simulink model "ES259A_BattVltgCorrln"  (R2013b)
settings: Solver=FixedStepDiscrete  SolverMode=SingleTasking  StartTime=0.0  StopTime=Inf  FixedStep=0.002  RelTol=1e-3
values from neighbouring files (symbols this model uses):
  BattVltgCorrlnAllwdVltgDif = DataDict.Calibration    [ES259A_BattVltgCorrln_DataDict.m]
  BattVltgCorrlnBattLoVltg = DataDict.Calibration    [ES259A_BattVltgCorrln_DataDict.m]
  BattVltgCorrlnBattOverVltg = DataDict.Calibration    [ES259A_BattVltgCorrln_DataDict.m]
  BattVltgCorrlnBattUnderVltg = DataDict.Calibration    [ES259A_BattVltgCorrln_DataDict.m]
  BattVltgCorrlnNtc0x03C0x0440x04CFailStep = DataDict.Calibration    [ES259A_BattVltgCorrln_DataDict.m]
  BattVltgCorrlnNtc0x03C0x0440x04CPassStep = DataDict.Calibration    [ES259A_BattVltgCorrln_DataDict.m]
  BattVltgCorrlnNtc0x03DFailStep = DataDict.Calibration    [ES259A_BattVltgCorrln_DataDict.m]
  BattVltgCorrlnNtc0x03DPassStep = DataDict.Calibration    [ES259A_BattVltgCorrln_DataDict.m]
  BattVltgCorrlnNtc0x0B0FailStep = DataDict.Calibration    [ES259A_BattVltgCorrln_DataDict.m]
  BattVltgCorrlnNtc0x0B0PassStep = DataDict.Calibration    [ES259A_BattVltgCorrln_DataDict.m]
  BattVltgCorrlnNtc0x0B1FailStep = DataDict.Calibration    [ES259A_BattVltgCorrln_DataDict.m]
  BattVltgCorrlnNtc0x0B1PassStep = DataDict.Calibration    [ES259A_BattVltgCorrln_DataDict.m]
  BattVltgCorrlnNtc0x0B5FailStep = DataDict.Calibration    [ES259A_BattVltgCorrln_DataDict.m]
  BattVltgCorrlnNtc0x0B5PassStep = DataDict.Calibration    [ES259A_BattVltgCorrln_DataDict.m]
  BattVltgCorrlnRcvrlBattLoVltg = DataDict.Calibration    [ES259A_BattVltgCorrln_DataDict.m]
  BattVltgCorrlnRcvrlBattOverVltg = DataDict.Calibration    [ES259A_BattVltgCorrln_DataDict.m]
  BattVltgCorrlnRcvrlBattUnderVltg = DataDict.Calibration    [ES259A_BattVltgCorrln_DataDict.m]
  BattVltgCorrlnSysMinVltg = DataDict.ImprtdCal    [ES250A_BattVltg_DataDict.m]    (also in ES259A_BattVltgCorrln_DataDict.m = DataDict.Calibration)
  BattVltgSwdMax = DataDict.Calibration    [ES250A_BattVltg_DataDict.m]
  ELECGLBPRM_STRTUPSTPWRDISCNCTBTESTCMPL_CNT_U08 = DataDict.Constant    [ES999A_ElecGlbPrm_DataDict.m]
  SYSVLTGFLTDUALIVTR_CNT_U08 = DataDict.Constant    [ES259A_BattVltgCorrln_DataDict.m]
undefined symbols (not defined in the file or in its folder): NtcNr1, NtcSts1, SigQlfr1
libraries: simulink x14
(part 6 of 7)

== system ES259A_BattVltgCorrln/BattVltgCorrln/BattVltgCorrlnPer1/WarmInit or Enable/Determine Independent Signals/Diagnose Inputs/NTC 3D/Pass NTC 3D/Copyright1 ==

== system ES259A_BattVltgCorrln/BattVltgCorrln/BattVltgCorrlnPer1/WarmInit or Enable/Determine Independent Signals/Diagnose Inputs/NTC 3D/Pass NTC 3D/SetNtcSts ==
  note: Only pass values 2 or 3 as input to NtcSts.
      | 2: PrePassd
      | 3: PreFaild
  NtcNr : Inport
  NtcStInfo : Inport  Port=2
  NtcSts : Inport  Port=3
  DebStep : Inport  Port=4
  Copyright1 : Subsystem  Description=|  mask(Copyright Information){none=on}
      | Copyright info block.                                               
      |                                                                     
      | Place copyright information at the top of every subsystem in design.
      mask prompts: none "No parameters"
      mask help: Place copyright information at the top of every subsystem in design.
      mask Display:
      | NxtrConf = 'Nexteer Confidential';
      | 
      | sys = bdroot; %handle for the current model ("system")
      | first = get_param(sys,'Created');
      | if(isempty(first))
      |     first = datestr(now,'yyyy');
      | else
      |     first = first(end-3:end);  %year is last four digits
      | end
      | 
      | last = get_param(sys,'LastModifiedDate');
      | if isempty(last)
      |     last = datestr(now,'yyyy');
      | else
      |     last = last(end-3:end);
      | end
      | 
      | if strcmp(first,last)
      |     fprintf('%s\nCopyright  %s Nexteer',NxtrConf,first);
      | else
      |     fprintf('%s\n%s%s-%s Nexteer',NxtrConf,char(169),first,last);
      | end
  Data Store Write1 : DataStoreWrite  RequirementInfo={} %GIDa_6d6848f0_15f2_42f8_b891_1052be6b64a1  DataStoreName=NtcQlfr3D
  ISO Fault Debounce Design NOT TO BE IMPLEMENTED IN THIS FDD USED ONLY FOR SIMULATION PURPOSES : Stateflow chart  TreatAsAtomicUnit=on
  Only here because I could not get model to run with enumerations in the stateflow diagram : DataTypeConversion  OutDataTypeStr=uint8
  Terminator : Terminator
  Terminator1 : Terminator
  wires:
  NtcStInfo/1 -> Terminator1/1
  NtcNr/1 -> Terminator/1
  NtcSts/1 -> Only here because I could not get model to run with enumerations in the stateflow diagram/1
  DebStep/1 -> ISO Fault Debounce Design NOT TO BE IMPLEMENTED IN THIS FDD USED ONLY FOR SIMULATION PURPOSES/2(DebStep)
  ISO Fault Debounce Design NOT TO BE IMPLEMENTED IN THIS FDD USED ONLY FOR SIMULATION PURPOSES/1(Qualifier) -> Data Store Write1/1
  Only here because I could not get model to run with enumerations in the stateflow diagram/1 -> ISO Fault Debounce Design NOT TO BE IMPLEMENTED IN THIS FDD USED ONLY FOR SIMULATION PURPOSES/1(NtcSts)

== system ES259A_BattVltgCorrln/BattVltgCorrln/BattVltgCorrlnPer1/WarmInit or Enable/Determine Independent Signals/Diagnose Inputs/NTC 44/GetNtcQlfrSts 0x044/Copyright1 ==

== system ES259A_BattVltgCorrln/BattVltgCorrln/BattVltgCorrlnPer1/WarmInit or Enable/Determine Independent Signals/Diagnose Inputs/NTC 44/GetNtcQlfrSts 0x044/GetNtcQlfrSts ==
  note: Enumeration of SigQlfr1
      |         SIGQLFR_NORES   (0)
      |         SIGQLFR_PASSD    (1)
      |         SIGQLFR_FAILD      (2)
  NtcNr : Inport
  CopyRight2 : Subsystem  Description=|  mask(Copyright Information){none=on}
      | Copyright info block.                                               
      |                                                                     
      | Place copyright information at the top of every subsystem in design.
      mask prompts: none "No parameters"
      mask help: Place copyright information at the top of every subsystem in design.
      mask Display:
      | NxtrConf = 'Nexteer Confidential';
      | 
      | sys = bdroot; %handle for the current model ("system")
      | first = get_param(sys,'Created');
      | first = first(end-3:end);  %year is last four digits
      | 
      | last = get_param(sys,'LastModifiedDate');
      | if isempty(last)
      |     last = datestr(now,'yyyy');
      | else
      |     last = last(end-3:end);
      | end
      | 
      | if strcmp(first,last)
      |     fprintf('%s -- Copyright %s Nexteer',NxtrConf,first)
      | else
      |     fprintf('%s -- %s%s- %s Nexteer',NxtrConf,char(169),first,last)
      | end
  Data Store Read5 : DataStoreRead  DataStoreName=NtcQlfr44
  Data Type Conversion : DataTypeConversion  OutDataTypeStr=uint8
  EOK : Constant  OutDataTypeStr=uint8
  Terminator : Terminator
  Return : Outport  InitialOutput=1
  Ntc0x044QlfrSts : Outport  Port=2
  wires:
  Data Store Read5/1 -> Data Type Conversion/1
  EOK/1 -> Return/1
  NtcNr/1 -> Terminator/1
  Data Type Conversion/1 -> Ntc0x044QlfrSts/1

== system ES259A_BattVltgCorrln/BattVltgCorrln/BattVltgCorrlnPer1/WarmInit or Enable/Determine Independent Signals/Diagnose Inputs/NTC 44/SetNtcSts 0x044/Copyright1 ==

== system ES259A_BattVltgCorrln/BattVltgCorrln/BattVltgCorrlnPer1/WarmInit or Enable/Determine Independent Signals/Diagnose Inputs/NTC 44/SetNtcSts 0x044/Do Nothing ==
  Action Port : ActionPort  ActionType=then
  Copyright1 : Subsystem  Description=|  mask(Copyright Information){none=on}
      | Copyright info block.                                               
      |                                                                     
      | Place copyright information at the top of every subsystem in design.
      mask prompts: none "No parameters"
      mask help: Place copyright information at the top of every subsystem in design.
      mask Display:
      | NxtrConf = 'Nexteer Confidential';
      | 
      | sys = bdroot; %handle for the current model ("system")
      | first = get_param(sys,'Created');
      | if(isempty(first))
      |     first = datestr(now,'yyyy');
      | else
      |     first = first(end-3:end);  %year is last four digits
      | end
      | 
      | last = get_param(sys,'LastModifiedDate');
      | if isempty(last)
      |     last = datestr(now,'yyyy');
      | else
      |     last = last(end-3:end);
      | end
      | 
      | if strcmp(first,last)
      |     fprintf('%s\nCopyright  %s Nexteer',NxtrConf,first);
      | else
      |     fprintf('%s\n%s%s-%s Nexteer',NxtrConf,char(169),first,last);
      | end

== system ES259A_BattVltgCorrln/BattVltgCorrln/BattVltgCorrlnPer1/WarmInit or Enable/Determine Independent Signals/Diagnose Inputs/NTC 44/SetNtcSts 0x044/Fails the test ==
  Action Port : ActionPort  ActionType=else
  BattVltgCorrlnNtc0x044FailStep : Constant  Value=BattVltgCorrlnNtc0x03C0x0440x04CFailStep
  Copyright1 : Subsystem  Description=|  mask(Copyright Information){none=on}
      | Copyright info block.                                               
      |                                                                     
      | Place copyright information at the top of every subsystem in design.
      mask prompts: none "No parameters"
      mask help: Place copyright information at the top of every subsystem in design.
      mask Display:
      | NxtrConf = 'Nexteer Confidential';
      | 
      | sys = bdroot; %handle for the current model ("system")
      | first = get_param(sys,'Created');
      | if(isempty(first))
      |     first = datestr(now,'yyyy');
      | else
      |     first = first(end-3:end);  %year is last four digits
      | end
      | 
      | last = get_param(sys,'LastModifiedDate');
      | if isempty(last)
      |     last = datestr(now,'yyyy');
      | else
      |     last = last(end-3:end);
      | end
      | 
      | if strcmp(first,last)
      |     fprintf('%s\nCopyright  %s Nexteer',NxtrConf,first);
      | else
      |     fprintf('%s\n%s%s-%s Nexteer',NxtrConf,char(169),first,last);
      | end
  Parameter Byte : Constant  OutDataTypeStr=uint8
  Status Type : Constant  Value=NtcSts1.NTCSTS_PREFAILD
  Ntc0x044 NtcStInfo : Outport
  Ntc0x044 NtcSts : Outport  Port=2
  Ntc0x044 FailStep : Outport  Port=3
  wires:
  Status Type/1 -> Ntc0x044 NtcSts/1
  BattVltgCorrlnNtc0x044FailStep/1 -> Ntc0x044 FailStep/1
  Parameter Byte/1 -> Ntc0x044 NtcStInfo/1

== system ES259A_BattVltgCorrln/BattVltgCorrln/BattVltgCorrlnPer1/WarmInit or Enable/Determine Independent Signals/Diagnose Inputs/NTC 44/SetNtcSts 0x044/Passes the test ==
  Action Port : ActionPort  ActionType=elseif
  BattVltgCorrlnNtc0x044PassStep : Constant  Value=BattVltgCorrlnNtc0x03C0x0440x04CPassStep
  Copyright1 : Subsystem  Description=|  mask(Copyright Information){none=on}
      | Copyright info block.                                               
      |                                                                     
      | Place copyright information at the top of every subsystem in design.
      mask prompts: none "No parameters"
      mask help: Place copyright information at the top of every subsystem in design.
      mask Display:
      | NxtrConf = 'Nexteer Confidential';
      | 
      | sys = bdroot; %handle for the current model ("system")
      | first = get_param(sys,'Created');
      | if(isempty(first))
      |     first = datestr(now,'yyyy');
      | else
      |     first = first(end-3:end);  %year is last four digits
      | end
      | 
      | last = get_param(sys,'LastModifiedDate');
      | if isempty(last)
      |     last = datestr(now,'yyyy');
      | else
      |     last = last(end-3:end);
      | end
      | 
      | if strcmp(first,last)
      |     fprintf('%s\nCopyright  %s Nexteer',NxtrConf,first);
      | else
      |     fprintf('%s\n%s%s-%s Nexteer',NxtrConf,char(169),first,last);
      | end
  Parameter Byte Data1 : Constant  Value=0  OutDataTypeStr=uint8
  Status Type : Constant  Value=NtcSts1.NTCSTS_PREPASSD
  Ntc0x044 NtcStInfo : Outport
  Ntc0x044 NtcSts : Outport  Port=2
  Ntc0x044 PassStep : Outport  Port=3
  wires:
  Status Type/1 -> Ntc0x044 NtcSts/1
  BattVltgCorrlnNtc0x044PassStep/1 -> Ntc0x044 PassStep/1
  Parameter Byte Data1/1 -> Ntc0x044 NtcStInfo/1

== system ES259A_BattVltgCorrln/BattVltgCorrln/BattVltgCorrlnPer1/WarmInit or Enable/Determine Independent Signals/Diagnose Inputs/NTC 44/SetNtcSts 0x044/SetNtcSts ==
  note: Only pass values 2 or 3 as input to NtcSts.
      | 2: PrePassd
      | 3: PreFaild
  NtcNr : Inport
  NtcStInfo : Inport  Port=2
  NtcSts : Inport  Port=3
  DebStep : Inport  Port=4
  Copyright1 : Subsystem  Description=|  mask(Copyright Information){none=on}
      | Copyright info block.                                               
      |                                                                     
      | Place copyright information at the top of every subsystem in design.
      mask prompts: none "No parameters"
      mask help: Place copyright information at the top of every subsystem in design.
      mask Display:
      | NxtrConf = 'Nexteer Confidential';
      | 
      | sys = bdroot; %handle for the current model ("system")
      | first = get_param(sys,'Created');
      | if(isempty(first))
      |     first = datestr(now,'yyyy');
      | else
      |     first = first(end-3:end);  %year is last four digits
      | end
      | 
      | last = get_param(sys,'LastModifiedDate');
      | if isempty(last)
      |     last = datestr(now,'yyyy');
      | else
      |     last = last(end-3:end);
      | end
      | 
      | if strcmp(first,last)
      |     fprintf('%s\nCopyright  %s Nexteer',NxtrConf,first);
      | else
      |     fprintf('%s\n%s%s-%s Nexteer',NxtrConf,char(169),first,last);
      | end
  Data Store Write1 : DataStoreWrite  RequirementInfo={} %GIDa_89fda807_da4f_4ef8_9f7d_e78b25b40171  DataStoreName=NtcQlfr44
  ISO Fault Debounce Design NOT TO BE IMPLEMENTED IN THIS FDD USED ONLY FOR SIMULATION PURPOSES : Stateflow chart  TreatAsAtomicUnit=on
  Only here because I could not get model to run with enumerations in the stateflow diagram : DataTypeConversion  OutDataTypeStr=uint8
  Terminator : Terminator
  Terminator1 : Terminator
  wires:
  NtcStInfo/1 -> Terminator1/1
  NtcNr/1 -> Terminator/1
  NtcSts/1 -> Only here because I could not get model to run with enumerations in the stateflow diagram/1
  DebStep/1 -> ISO Fault Debounce Design NOT TO BE IMPLEMENTED IN THIS FDD USED ONLY FOR SIMULATION PURPOSES/2(DebStep)
  Only here because I could not get model to run with enumerations in the stateflow diagram/1 -> ISO Fault Debounce Design NOT TO BE IMPLEMENTED IN THIS FDD USED ONLY FOR SIMULATION PURPOSES/1(NtcSts)
  ISO Fault Debounce Design NOT TO BE IMPLEMENTED IN THIS FDD USED ONLY FOR SIMULATION PURPOSES/1(Qualifier) -> Data Store Write1/1

== system ES259A_BattVltgCorrln/BattVltgCorrln/BattVltgCorrlnPer1/WarmInit or Enable/Determine Independent Signals/Diagnose Inputs/NTC 4C/GetNtcQlfrSts 0x04C/Copyright1 ==

== system ES259A_BattVltgCorrln/BattVltgCorrln/BattVltgCorrlnPer1/WarmInit or Enable/Determine Independent Signals/Diagnose Inputs/NTC 4C/GetNtcQlfrSts 0x04C/GetNtcQlfrSts ==
  note: Enumeration of SigQlfr1
      |         SIGQLFR_NORES   (0)
      |         SIGQLFR_PASSD    (1)
      |         SIGQLFR_FAILD      (2)
  NtcNr : Inport
  CopyRight2 : Subsystem  Description=|  mask(Copyright Information){none=on}
      | Copyright info block.                                               
      |                                                                     
      | Place copyright information at the top of every subsystem in design.
      mask prompts: none "No parameters"
      mask help: Place copyright information at the top of every subsystem in design.
      mask Display:
      | NxtrConf = 'Nexteer Confidential';
      | 
      | sys = bdroot; %handle for the current model ("system")
      | first = get_param(sys,'Created');
      | first = first(end-3:end);  %year is last four digits
      | 
      | last = get_param(sys,'LastModifiedDate');
      | if isempty(last)
      |     last = datestr(now,'yyyy');
      | else
      |     last = last(end-3:end);
      | end
      | 
      | if strcmp(first,last)
      |     fprintf('%s -- Copyright %s Nexteer',NxtrConf,first)
      | else
      |     fprintf('%s -- %s%s- %s Nexteer',NxtrConf,char(169),first,last)
      | end
  Data Store Read5 : DataStoreRead  DataStoreName=NtcQlfr4C
  Data Type Conversion : DataTypeConversion  OutDataTypeStr=uint8
  EOK : Constant  OutDataTypeStr=uint8
  Terminator : Terminator
  Return : Outport  InitialOutput=1
  Ntc0x04CQlfrSts : Outport  Port=2
  wires:
  Data Store Read5/1 -> Data Type Conversion/1
  EOK/1 -> Return/1
  NtcNr/1 -> Terminator/1
  Data Type Conversion/1 -> Ntc0x04CQlfrSts/1

== system ES259A_BattVltgCorrln/BattVltgCorrln/BattVltgCorrlnPer1/WarmInit or Enable/Determine Independent Signals/Diagnose Inputs/NTC 4C/SetNtcSts 0x04C/Copyright1 ==

== system ES259A_BattVltgCorrln/BattVltgCorrln/BattVltgCorrlnPer1/WarmInit or Enable/Determine Independent Signals/Diagnose Inputs/NTC 4C/SetNtcSts 0x04C/Do Nothing ==
  Action Port : ActionPort  ActionType=then
  Copyright1 : Subsystem  Description=|  mask(Copyright Information){none=on}
      | Copyright info block.                                               
      |                                                                     
      | Place copyright information at the top of every subsystem in design.
      mask prompts: none "No parameters"
      mask help: Place copyright information at the top of every subsystem in design.
      mask Display:
      | NxtrConf = 'Nexteer Confidential';
      | 
      | sys = bdroot; %handle for the current model ("system")
      | first = get_param(sys,'Created');
      | if(isempty(first))
      |     first = datestr(now,'yyyy');
      | else
      |     first = first(end-3:end);  %year is last four digits
      | end
      | 
      | last = get_param(sys,'LastModifiedDate');
      | if isempty(last)
      |     last = datestr(now,'yyyy');
      | else
      |     last = last(end-3:end);
      | end
      | 
      | if strcmp(first,last)
      |     fprintf('%s\nCopyright  %s Nexteer',NxtrConf,first);
      | else
      |     fprintf('%s\n%s%s-%s Nexteer',NxtrConf,char(169),first,last);
      | end

== system ES259A_BattVltgCorrln/BattVltgCorrln/BattVltgCorrlnPer1/WarmInit or Enable/Determine Independent Signals/Diagnose Inputs/NTC 4C/SetNtcSts 0x04C/Fails the test ==
  Action Port : ActionPort  ActionType=else
  BattVltgCorrlnNtc0x04CFailStep : Constant  Value=BattVltgCorrlnNtc0x03C0x0440x04CFailStep
  Copyright1 : Subsystem  Description=|  mask(Copyright Information){none=on}
      | Copyright info block.                                               
      |                                                                     
      | Place copyright information at the top of every subsystem in design.
      mask prompts: none "No parameters"
      mask help: Place copyright information at the top of every subsystem in design.
      mask Display:
      | NxtrConf = 'Nexteer Confidential';
      | 
      | sys = bdroot; %handle for the current model ("system")
      | first = get_param(sys,'Created');
      | if(isempty(first))
      |     first = datestr(now,'yyyy');
      | else
      |     first = first(end-3:end);  %year is last four digits
      | end
      | 
      | last = get_param(sys,'LastModifiedDate');
      | if isempty(last)
      |     last = datestr(now,'yyyy');
      | else
      |     last = last(end-3:end);
      | end
      | 
      | if strcmp(first,last)
      |     fprintf('%s\nCopyright  %s Nexteer',NxtrConf,first);
      | else
      |     fprintf('%s\n%s%s-%s Nexteer',NxtrConf,char(169),first,last);
      | end
  Parameter Byte : Constant  OutDataTypeStr=uint8
  Status Type : Constant  Value=NtcSts1.NTCSTS_PREFAILD
  Ntc0x04C NtcStInfo : Outport
  Ntc0x04C NtcSts : Outport  Port=2
  Ntc0x04C PassStep : Outport  Port=3
  wires:
  Status Type/1 -> Ntc0x04C NtcSts/1
  Parameter Byte/1 -> Ntc0x04C NtcStInfo/1
  BattVltgCorrlnNtc0x04CFailStep/1 -> Ntc0x04C PassStep/1

== system ES259A_BattVltgCorrln/BattVltgCorrln/BattVltgCorrlnPer1/WarmInit or Enable/Determine Independent Signals/Diagnose Inputs/NTC 4C/SetNtcSts 0x04C/Passes the test ==
  Action Port : ActionPort  ActionType=elseif
  BattVltgCorrlnNtc0x04CPassStep : Constant  Value=BattVltgCorrlnNtc0x03C0x0440x04CPassStep
  Copyright1 : Subsystem  Description=|  mask(Copyright Information){none=on}
      | Copyright info block.                                               
      |                                                                     
      | Place copyright information at the top of every subsystem in design.
      mask prompts: none "No parameters"
      mask help: Place copyright information at the top of every subsystem in design.
      mask Display:
      | NxtrConf = 'Nexteer Confidential';
      | 
      | sys = bdroot; %handle for the current model ("system")
      | first = get_param(sys,'Created');
      | if(isempty(first))
      |     first = datestr(now,'yyyy');
      | else
      |     first = first(end-3:end);  %year is last four digits
      | end
      | 
      | last = get_param(sys,'LastModifiedDate');
      | if isempty(last)
      |     last = datestr(now,'yyyy');
      | else
      |     last = last(end-3:end);
      | end
      | 
      | if strcmp(first,last)
      |     fprintf('%s\nCopyright  %s Nexteer',NxtrConf,first);
      | else
      |     fprintf('%s\n%s%s-%s Nexteer',NxtrConf,char(169),first,last);
      | end
  Parameter Byte Data1 : Constant  Value=0  OutDataTypeStr=uint8
  Status Type : Constant  Value=NtcSts1.NTCSTS_PREPASSD
  Ntc0x04C NtcStInfo : Outport
  Ntc0x04C NtcSts : Outport  Port=2
  Ntc0x04C PassStep : Outport  Port=3
  wires:
  Status Type/1 -> Ntc0x04C NtcSts/1
  Parameter Byte Data1/1 -> Ntc0x04C NtcStInfo/1
  BattVltgCorrlnNtc0x04CPassStep/1 -> Ntc0x04C PassStep/1

== system ES259A_BattVltgCorrln/BattVltgCorrln/BattVltgCorrlnPer1/WarmInit or Enable/Determine Independent Signals/Diagnose Inputs/NTC 4C/SetNtcSts 0x04C/SetNtcSts ==
  note: Only pass values 2 or 3 as input to NtcSts.
      | 2: PrePassd
      | 3: PreFaild
  NtcNr : Inport
  NtcStInfo : Inport  Port=2
  NtcSts : Inport  Port=3
  DebStep : Inport  Port=4
  Copyright1 : Subsystem  Description=|  mask(Copyright Information){none=on}
      | Copyright info block.                                               
      |                                                                     
      | Place copyright information at the top of every subsystem in design.
      mask prompts: none "No parameters"
      mask help: Place copyright information at the top of every subsystem in design.
      mask Display:
      | NxtrConf = 'Nexteer Confidential';
      | 
      | sys = bdroot; %handle for the current model ("system")
      | first = get_param(sys,'Created');
      | if(isempty(first))
      |     first = datestr(now,'yyyy');
      | else
      |     first = first(end-3:end);  %year is last four digits
      | end
      | 
      | last = get_param(sys,'LastModifiedDate');
      | if isempty(last)
      |     last = datestr(now,'yyyy');
      | else
      |     last = last(end-3:end);
      | end
      | 
      | if strcmp(first,last)
      |     fprintf('%s\nCopyright  %s Nexteer',NxtrConf,first);
      | else
      |     fprintf('%s\n%s%s-%s Nexteer',NxtrConf,char(169),first,last);
      | end
  Data Store Write1 : DataStoreWrite  RequirementInfo={} %GIDa_0b6832db_b5ce_44a6_8c80_102ac06d195d  DataStoreName=NtcQlfr4C
  ISO Fault Debounce Design NOT TO BE IMPLEMENTED IN THIS FDD USED ONLY FOR SIMULATION PURPOSES : Stateflow chart  TreatAsAtomicUnit=on
  Only here because I could not get model to run with enumerations in the stateflow diagram : DataTypeConversion  OutDataTypeStr=uint8
  Terminator : Terminator
  Terminator1 : Terminator
  wires:
  NtcStInfo/1 -> Terminator1/1
  NtcNr/1 -> Terminator/1
  NtcSts/1 -> Only here because I could not get model to run with enumerations in the stateflow diagram/1
  DebStep/1 -> ISO Fault Debounce Design NOT TO BE IMPLEMENTED IN THIS FDD USED ONLY FOR SIMULATION PURPOSES/2(DebStep)
  Only here because I could not get model to run with enumerations in the stateflow diagram/1 -> ISO Fault Debounce Design NOT TO BE IMPLEMENTED IN THIS FDD USED ONLY FOR SIMULATION PURPOSES/1(NtcSts)
  ISO Fault Debounce Design NOT TO BE IMPLEMENTED IN THIS FDD USED ONLY FOR SIMULATION PURPOSES/1(Qualifier) -> Data Store Write1/1

== system ES259A_BattVltgCorrln/BattVltgCorrln/BattVltgCorrlnPer1/WarmInit or Enable/Instantaneous Correlation/Correlation Check/BattVltg vs BattVltgSwd1/BattVltg <= 16/Copyright1 ==

== system ES259A_BattVltgCorrln/BattVltgCorrln/BattVltgCorrlnPer1/WarmInit or Enable/Instantaneous Correlation/Correlation Check/BattVltg vs BattVltgSwd1/BattVltg > 16/Copyright1 ==

== system ES259A_BattVltgCorrln/BattVltgCorrln/BattVltgCorrlnPer1/WarmInit or Enable/Instantaneous Correlation/Correlation Check/BattVltgSwd2 vs BattVltg/BattVltg <= 16/Copyright1 ==

== system ES259A_BattVltgCorrln/BattVltgCorrln/BattVltgCorrlnPer1/WarmInit or Enable/Instantaneous Correlation/Correlation Check/BattVltgSwd2 vs BattVltg/BattVltg > 16/Copyright1 ==

== system ES259A_BattVltgCorrln/BattVltgCorrln/BattVltgCorrlnPer1/WarmInit or Enable/Determine Independent Signals/Diagnose Inputs/NTC 3C/SetNtcSts 0x03C/Fails the test/Copyright1 ==

== system ES259A_BattVltgCorrln/BattVltgCorrln/BattVltgCorrlnPer1/WarmInit or Enable/Determine Independent Signals/Diagnose Inputs/NTC 3C/SetNtcSts 0x03C/Passes the test/Copyright1 ==

== system ES259A_BattVltgCorrln/BattVltgCorrln/BattVltgCorrlnPer1/WarmInit or Enable/Determine Independent Signals/Diagnose Inputs/NTC 3C/SetNtcSts 0x03C/SetNtcSts/Copyright1 ==

== system ES259A_BattVltgCorrln/BattVltgCorrln/BattVltgCorrlnPer1/WarmInit or Enable/Determine Independent Signals/Diagnose Inputs/NTC 3D/Fail NTC 3D/SetNtcSts/Copyright1 ==

== system ES259A_BattVltgCorrln/BattVltgCorrln/BattVltgCorrlnPer1/WarmInit or Enable/Determine Independent Signals/Diagnose Inputs/NTC 3D/Pass NTC 3D/SetNtcSts/Copyright1 ==

== system ES259A_BattVltgCorrln/BattVltgCorrln/BattVltgCorrlnPer1/WarmInit or Enable/Determine Independent Signals/Diagnose Inputs/NTC 44/GetNtcQlfrSts 0x044/GetNtcQlfrSts/CopyRight2 ==

== system ES259A_BattVltgCorrln/BattVltgCorrln/BattVltgCorrlnPer1/WarmInit or Enable/Determine Independent Signals/Diagnose Inputs/NTC 44/SetNtcSts 0x044/Do Nothing/Copyright1 ==

== system ES259A_BattVltgCorrln/BattVltgCorrln/BattVltgCorrlnPer1/WarmInit or Enable/Determine Independent Signals/Diagnose Inputs/NTC 44/SetNtcSts 0x044/Fails the test/Copyright1 ==

== system ES259A_BattVltgCorrln/BattVltgCorrln/BattVltgCorrlnPer1/WarmInit or Enable/Determine Independent Signals/Diagnose Inputs/NTC 44/SetNtcSts 0x044/Passes the test/Copyright1 ==

== system ES259A_BattVltgCorrln/BattVltgCorrln/BattVltgCorrlnPer1/WarmInit or Enable/Determine Independent Signals/Diagnose Inputs/NTC 44/SetNtcSts 0x044/SetNtcSts/Copyright1 ==

== system ES259A_BattVltgCorrln/BattVltgCorrln/BattVltgCorrlnPer1/WarmInit or Enable/Determine Independent Signals/Diagnose Inputs/NTC 4C/GetNtcQlfrSts 0x04C/GetNtcQlfrSts/CopyRight2 ==

== system ES259A_BattVltgCorrln/BattVltgCorrln/BattVltgCorrlnPer1/WarmInit or Enable/Determine Independent Signals/Diagnose Inputs/NTC 4C/SetNtcSts 0x04C/Do Nothing/Copyright1 ==

== system ES259A_BattVltgCorrln/BattVltgCorrln/BattVltgCorrlnPer1/WarmInit or Enable/Determine Independent Signals/Diagnose Inputs/NTC 4C/SetNtcSts 0x04C/Fails the test/Copyright1 ==

== system ES259A_BattVltgCorrln/BattVltgCorrln/BattVltgCorrlnPer1/WarmInit or Enable/Determine Independent Signals/Diagnose Inputs/NTC 4C/SetNtcSts 0x04C/Passes the test/Copyright1 ==

== system ES259A_BattVltgCorrln/BattVltgCorrln/BattVltgCorrlnPer1/WarmInit or Enable/Determine Independent Signals/Diagnose Inputs/NTC 4C/SetNtcSts 0x04C/SetNtcSts/Copyright1 ==

== stateflow chart ES259A_BattVltgCorrln/BattVltgCorrln/BattVltgCorrlnPer1/WarmInit or Enable/Determine Independent Signals/Diagnose Inputs/NTC 44/SetNtcSts 0x044/SetNtcSts/ISO Fault Debounce Design NOT TO BE IMPLEMENTED IN THIS FDD USED ONLY FOR SIMULATION PURPOSES ==
  note: NTCSTS_PASSD           (0)
      | NTCSTS_FAILD             (1)
      | NTCSTS_PREPASSD   (2)
      | NTCSTS_PREFAILD     (3)
      |
      | SIGQLFR_NORES        (0)
      | SIGQLFR_PASSD         (1)
      | SIGQLFR_FAILD           (2)
  note: Fail step Loop
  note: Pass step Loop
  note: 
  (default) -> (junction 89)
  (junction 89) -> (junction 95) [order 1] : [NtcSts == 3]
  (junction 89) -> (junction 93) [order 2] : [ NtcSts == 2]
  (junction 93) -> (junction 230) [order 2] : {
      | DebCntr = DebCntr - DebStep;
      | }
  (junction 95) -> (junction 216) [order 2] : [DebCntr <= 0]
      | {
      | DebCntr = DebStep;
      | }
  (junction 95) -> (junction 103) [order 1] : [DebCntr > 0]
  (junction 93) -> (junction 123) [order 1] : [(DebCntr - DebStep) <= -32768]
      | {
      | DebCntr = -32768;
      | Qualifier = 1;
      | }
  (junction 230) -> (junction 231)
  (junction 103) -> (junction 216) [order 2] : {
      | DebCntr = DebCntr + DebStep;
      | }
  (junction 216) -> (junction 220) [order 2]
  (junction 216) -> (junction 220) [order 1] : [(DebCntr + DebStep) >=32767]
      | {
      | DebCntr = 32767;
      | Qualifier =2;
      | }
  (junction 103) -> (junction 220) [order 1] : [(DebCntr + DebStep) >=32767]
      | {
      | DebCntr = 32767;
      | Qualifier =2;
      | }
  (junction 220) -> (junction 141)
  (junction 123) -> (junction 141)
  (junction 231) -> (junction 123)
  (junction 141) -> (junction 159)
  data: NtcSts input uint8; Qualifier output uint8 =0; DebStep input uint16; DebCntr local int16

== matlab function ES259A_BattVltgCorrln/BattVltgCorrln/BattVltgCorrlnPer1/WarmInit or Enable/Instantaneous Correlation/Correlation Check/TestOk TruthTable ==
  data: BattVltgvsBattVltgSwd1 input boolean; BattVltgOk output uint8; BattVltgSwd1vsBattVltgSwd2 input boolean; BattVltgSwd2vsBattVltg input boolean; BattVltgSwd1Ok output uint8; BattVltgSwd2Ok output uint8
function [BattVltgOk, BattVltgSwd1Ok, BattVltgSwd2Ok] = fcn(BattVltgvsBattVltgSwd1, BattVltgSwd1vsBattVltgSwd2, BattVltgSwd2vsBattVltg)

aVarTruthTableCondition_1 = false;
aVarTruthTableCondition_2 = false;
aVarTruthTableCondition_3 = false;


% BattVltgvsBattVltgSwd1 TestOk

aVarTruthTableCondition_1 = logical(BattVltgvsBattVltgSwd1 == 1);

% BattVltgSwd1vsBattVltgSwd2 TestOk

aVarTruthTableCondition_2 = logical(BattVltgSwd1vsBattVltgSwd2 == 1);

% BattVltgSwd2vsBattVltg TestOk

aVarTruthTableCondition_3 = logical(BattVltgSwd2vsBattVltg == 1);

if (aVarTruthTableCondition_1 && aVarTruthTableCondition_2 && aVarTruthTableCondition_3)
    aFcnTruthTableAction_1();
elseif (aVarTruthTableCondition_1 && aVarTruthTableCondition_2 && ~aVarTruthTableCondition_3)
    aFcnTruthTableAction_1();
elseif (aVarTruthTableCondition_1 && ~aVarTruthTableCondition_2 && aVarTruthTableCondition_3)
    aFcnTruthTableAction_1();
elseif (aVarTruthTableCondition_1 && ~aVarTruthTableCondition_2 && ~aVarTruthTableCondition_3)
    aFcnTruthTableAction_2();
elseif (~aVarTruthTableCondition_1 && aVarTruthTableCondition_2 && aVarTruthTableCondition_3)
    aFcnTruthTableAction_1();
elseif (~aVarTruthTableCondition_1 && aVarTruthTableCondition_2 && ~aVarTruthTableCondition_3)
    aFcnTruthTableAction_4();
elseif (~aVarTruthTableCondition_1 && ~aVarTruthTableCondition_2 && aVarTruthTableCondition_3)
    aFcnTruthTableAction_3();
else % Default
    aFcnTruthTableAction_5();
end

function aFcnTruthTableAction_1()

% All good

BattVltgOk = uint8(1);
BattVltgSwd1Ok = uint8(1);
BattVltgSwd2Ok = uint8(1);

function aFcnTruthTableAction_2()

% BattVltgSwd2 bad

BattVltgOk = uint8(1);
BattVltgSwd1Ok = uint8(1);
BattVltgSwd2Ok = uint8(0);

function aFcnTruthTableAction_3()

% BattVltgSwd1 bad

BattVltgOk = uint8(1);
BattVltgSwd1Ok = uint8(0);
BattVltgSwd2Ok = uint8(1);

function aFcnTruthTableAction_4()

% BattVltg bad

BattVltgOk = uint8(0);
BattVltgSwd1Ok = uint8(1);
BattVltgSwd2Ok = uint8(1);

function aFcnTruthTableAction_5()

% All bad

BattVltgOk = uint8(0);
BattVltgSwd1Ok = uint8(0);
BattVltgSwd2Ok = uint8(0);

== stateflow chart ES259A_BattVltgCorrln/BattVltgCorrln/BattVltgCorrlnPer1/WarmInit or Enable/Determine Independent Signals/Diagnose Inputs/NTC 4C/SetNtcSts 0x04C/SetNtcSts/ISO Fault Debounce Design NOT TO BE IMPLEMENTED IN THIS FDD USED ONLY FOR SIMULATION PURPOSES ==
  note: NTCSTS_PASSD           (0)
      | NTCSTS_FAILD             (1)
      | NTCSTS_PREPASSD   (2)
      | NTCSTS_PREFAILD     (3)
      |
      | SIGQLFR_NORES        (0)
      | SIGQLFR_PASSD         (1)
      | SIGQLFR_FAILD           (2)
  note: Fail step Loop
  note: Pass step Loop
  note: 
  (default) -> (junction 89)
  (junction 89) -> (junction 95) [order 1] : [NtcSts == 3]
  (junction 89) -> (junction 93) [order 2] : [ NtcSts == 2]
  (junction 93) -> (junction 230) [order 2] : {
      | DebCntr = DebCntr - DebStep;
      | }
  (junction 95) -> (junction 216) [order 2] : [DebCntr <= 0]
      | {
      | DebCntr = DebStep;
      | }
  (junction 95) -> (junction 103) [order 1] : [DebCntr > 0]
  (junction 93) -> (junction 123) [order 1] : [(DebCntr - DebStep) <= -32768]
      | {
      | DebCntr = -32768;
      | Qualifier = 1;
      | }
  (junction 230) -> (junction 231)
  (junction 103) -> (junction 216) [order 2] : {
      | DebCntr = DebCntr + DebStep;
      | }
  (junction 216) -> (junction 220) [order 2]
  (junction 216) -> (junction 220) [order 1] : [(DebCntr + DebStep) >=32767]
      | {
      | DebCntr = 32767;
      | Qualifier =2;
      | }
  (junction 103) -> (junction 220) [order 1] : [(DebCntr + DebStep) >=32767]
      | {
      | DebCntr = 32767;
      | Qualifier =2;
      | }
  (junction 220) -> (junction 141)
  (junction 123) -> (junction 141)
  (junction 231) -> (junction 123)
  (junction 141) -> (junction 159)
  data: NtcSts input uint8; Qualifier output uint8 =0; DebStep input uint16; DebCntr local int16

== stateflow chart ES259A_BattVltgCorrln/BattVltgCorrln/BattVltgCorrlnPer1/WarmInit or Enable/Determine Independent Signals/Diagnose Inputs/NTC 3C/SetNtcSts 0x03C/SetNtcSts/ISO Fault Debounce Design NOT TO BE IMPLEMENTED IN THIS FDD USED ONLY FOR SIMULATION PURPOSES ==
  note: NTCSTS_PASSD           (0)
      | NTCSTS_FAILD             (1)
      | NTCSTS_PREPASSD   (2)
      | NTCSTS_PREFAILD     (3)
      |
      | SIGQLFR_NORES        (0)
      | SIGQLFR_PASSD         (1)
      | SIGQLFR_FAILD           (2)
  note: Fail step Loop
  note: Pass step Loop
  note: 
  (default) -> (junction 89)
  (junction 89) -> (junction 95) [order 1] : [NtcSts == 3]
  (junction 89) -> (junction 93) [order 2] : [ NtcSts == 2]
  (junction 93) -> (junction 230) [order 2] : {
      | DebCntr = DebCntr - DebStep;
      | }
  (junction 95) -> (junction 216) [order 2] : [DebCntr <= 0]
      | {
      | DebCntr = DebStep;
      | }
  (junction 95) -> (junction 103) [order 1] : [DebCntr > 0]
  (junction 93) -> (junction 123) [order 1] : [(DebCntr - DebStep) <= -32768]
      | {
      | DebCntr = -32768;
      | Qualifier = 1;
      | }
  (junction 230) -> (junction 231)
  (junction 103) -> (junction 216) [order 2] : {
      | DebCntr = DebCntr + DebStep;
      | }
  (junction 216) -> (junction 220) [order 2]
  (junction 216) -> (junction 220) [order 1] : [(DebCntr + DebStep) >=32767]
      | {
      | DebCntr = 32767;
      | Qualifier =2;
      | }
  (junction 103) -> (junction 220) [order 1] : [(DebCntr + DebStep) >=32767]
      | {
      | DebCntr = 32767;
      | Qualifier =2;
      | }
  (junction 220) -> (junction 141)
  (junction 123) -> (junction 141)
  (junction 231) -> (junction 123)
  (junction 141) -> (junction 159)
  data: NtcSts input uint8; Qualifier output uint8 =0; DebStep input uint16; DebCntr local int16

== stateflow chart ES259A_BattVltgCorrln/BattVltgCorrln/BattVltgCorrlnPer1/WarmInit or Enable/Determine Independent Signals/Diagnose Inputs/NTC 3D/Fail NTC 3D/SetNtcSts/ISO Fault Debounce Design NOT TO BE IMPLEMENTED IN THIS FDD USED ONLY FOR SIMULATION PURPOSES ==
  note: NTCSTS_PASSD           (0)
      | NTCSTS_FAILD             (1)
      | NTCSTS_PREPASSD   (2)
      | NTCSTS_PREFAILD     (3)
      |
      | SIGQLFR_NORES        (0)
      | SIGQLFR_PASSD         (1)
      | SIGQLFR_FAILD           (2)
  note: Fail step Loop
  note: Pass step Loop
  note: 
  (default) -> (junction 89)
  (junction 89) -> (junction 95) [order 1] : [NtcSts == 3]
  (junction 89) -> (junction 93) [order 2] : [ NtcSts == 2]
  (junction 93) -> (junction 230) [order 2] : {
      | DebCntr = DebCntr - DebStep;
      | }
  (junction 95) -> (junction 216) [order 2] : [DebCntr <= 0]
      | {
      | DebCntr = DebStep;
      | }
  (junction 95) -> (junction 103) [order 1] : [DebCntr > 0]
  (junction 93) -> (junction 123) [order 1] : [(DebCntr - DebStep) <= -32768]
      | {
      | DebCntr = -32768;
      | Qualifier = 1;
      | }
  (junction 230) -> (junction 231)
  (junction 103) -> (junction 216) [order 2] : {
      | DebCntr = DebCntr + DebStep;
      | }
  (junction 216) -> (junction 220) [order 2]
  (junction 216) -> (junction 220) [order 1] : [(DebCntr + DebStep) >=32767]
      | {
      | DebCntr = 32767;
      | Qualifier =2;
      | }
  (junction 103) -> (junction 220) [order 1] : [(DebCntr + DebStep) >=32767]
      | {
      | DebCntr = 32767;
      | Qualifier =2;
      | }
  (junction 220) -> (junction 141)
  (junction 123) -> (junction 141)
  (junction 231) -> (junction 123)
  (junction 141) -> (junction 159)
  data: NtcSts input uint8; Qualifier output uint8 =0; DebStep input uint16; DebCntr local int16

== stateflow chart ES259A_BattVltgCorrln/BattVltgCorrln/BattVltgCorrlnPer1/Battery Voltage Diagnostics/Inhibition Off/BattVltg > OverVltg/SetNtcStsB0/ISO Fault Debounce Design NOT TO BE IMPLEMENTED IN THIS FDD USED ONLY FOR SIMULATION PURPOSES ==
  note: NTCSTS_PASSD           (0)
      | NTCSTS_FAILD             (1)
      | NTCSTS_PREPASSD   (2)
      | NTCSTS_PREFAILD     (3)
      |
      | SIGQLFR_NORES        (0)
      | SIGQLFR_PASSD         (1)
      | SIGQLFR_FAILD           (2)
  note: Fail step Loop
  note: Pass step Loop
  note: 
  (default) -> (junction 89)
  (junction 89) -> (junction 95) [order 1] : [NtcSts == 3]
  (junction 89) -> (junction 93) [order 2] : [ NtcSts == 2]
  (junction 93) -> (junction 230) [order 2] : {
      | DebCntr = DebCntr - DebStep;
      | }
  (junction 95) -> (junction 216) [order 2] : [DebCntr <= 0]
      | {
      | DebCntr = DebStep;
      | }
  (junction 95) -> (junction 103) [order 1] : [DebCntr > 0]
  (junction 93) -> (junction 123) [order 1] : [(DebCntr - DebStep) <= -32768]
      | {
      | DebCntr = -32768;
      | Qualifier = 1;
      | }
  (junction 230) -> (junction 231)
  (junction 103) -> (junction 216) [order 2] : {
      | DebCntr = DebCntr + DebStep;
      | }
  (junction 216) -> (junction 220) [order 2]
  (junction 216) -> (junction 220) [order 1] : [(DebCntr + DebStep) >=32767]
      | {
      | DebCntr = 32767;
      | Qualifier =2;
      | }
  (junction 103) -> (junction 220) [order 1] : [(DebCntr + DebStep) >=32767]
      | {
      | DebCntr = 32767;
      | Qualifier =2;
      | }
  (junction 220) -> (junction 141)
  (junction 123) -> (junction 141)
  (junction 231) -> (junction 123)
  (junction 141) -> (junction 159)
  data: NtcSts input uint8; Qualifier output uint8 =0; DebStep input uint16; DebCntr local int16

== stateflow chart ES259A_BattVltgCorrln/BattVltgCorrln/BattVltgCorrlnPer1/WarmInit or Enable/Determine Independent Signals/Diagnose Inputs/NTC 3D/Pass NTC 3D/SetNtcSts/ISO Fault Debounce Design NOT TO BE IMPLEMENTED IN THIS FDD USED ONLY FOR SIMULATION PURPOSES ==
  note: NTCSTS_PASSD           (0)
      | NTCSTS_FAILD             (1)
      | NTCSTS_PREPASSD   (2)
      | NTCSTS_PREFAILD     (3)
      |
      | SIGQLFR_NORES        (0)
      | SIGQLFR_PASSD         (1)
      | SIGQLFR_FAILD           (2)
  note: Fail step Loop
  note: Pass step Loop
  note: 
  (default) -> (junction 89)
  (junction 89) -> (junction 95) [order 1] : [NtcSts == 3]
  (junction 89) -> (junction 93) [order 2] : [ NtcSts == 2]
  (junction 93) -> (junction 230) [order 2] : {
      | DebCntr = DebCntr - DebStep;
      | }
  (junction 95) -> (junction 216) [order 2] : [DebCntr <= 0]
      | {
      | DebCntr = DebStep;
      | }
  (junction 95) -> (junction 103) [order 1] : [DebCntr > 0]
  (junction 93) -> (junction 123) [order 1] : [(DebCntr - DebStep) <= -32768]
      | {
      | DebCntr = -32768;
      | Qualifier = 1;
      | }
  (junction 230) -> (junction 231)
  (junction 103) -> (junction 216) [order 2] : {
      | DebCntr = DebCntr + DebStep;
      | }
  (junction 216) -> (junction 220) [order 2]
  (junction 216) -> (junction 220) [order 1] : [(DebCntr + DebStep) >=32767]
      | {
      | DebCntr = 32767;
      | Qualifier =2;
      | }
  (junction 103) -> (junction 220) [order 1] : [(DebCntr + DebStep) >=32767]
      | {
      | DebCntr = 32767;
      | Qualifier =2;
      | }
  (junction 220) -> (junction 141)
  (junction 123) -> (junction 141)
  (junction 231) -> (junction 123)
  (junction 141) -> (junction 159)
  data: NtcSts input uint8; Qualifier output uint8 =0; DebStep input uint16; DebCntr local int16

== stateflow chart ES259A_BattVltgCorrln/BattVltgCorrln/BattVltgCorrlnPer1/Battery Voltage Diagnostics/Inhibition Off/BattVltg > OverVltg/SetNtcStsB1/ISO Fault Debounce Design NOT TO BE IMPLEMENTED IN THIS FDD USED ONLY FOR SIMULATION PURPOSES ==
  note: NTCSTS_PASSD           (0)
      | NTCSTS_FAILD             (1)
      | NTCSTS_PREPASSD   (2)
      | NTCSTS_PREFAILD     (3)
      |
      | SIGQLFR_NORES        (0)
      | SIGQLFR_PASSD         (1)
      | SIGQLFR_FAILD           (2)
  note: Fail step Loop
  note: Pass step Loop
  note: 
  (default) -> (junction 89)
  (junction 89) -> (junction 95) [order 1] : [NtcSts == 3]
  (junction 89) -> (junction 93) [order 2] : [ NtcSts == 2]
  (junction 93) -> (junction 230) [order 2] : {
      | DebCntr = DebCntr - DebStep;
      | }
  (junction 95) -> (junction 216) [order 2] : [DebCntr <= 0]
      | {
      | DebCntr = DebStep;
      | }
  (junction 95) -> (junction 103) [order 1] : [DebCntr > 0]
  (junction 93) -> (junction 123) [order 1] : [(DebCntr - DebStep) <= -32768]
      | {
      | DebCntr = -32768;
      | Qualifier = 1;
      | }
  (junction 230) -> (junction 231)
  (junction 103) -> (junction 216) [order 2] : {
      | DebCntr = DebCntr + DebStep;
      | }
  (junction 216) -> (junction 220) [order 2]
  (junction 216) -> (junction 220) [order 1] : [(DebCntr + DebStep) >=32767]
      | {
      | DebCntr = 32767;
      | Qualifier =2;
      | }
  (junction 103) -> (junction 220) [order 1] : [(DebCntr + DebStep) >=32767]
      | {
      | DebCntr = 32767;
      | Qualifier =2;
      | }
  (junction 220) -> (junction 141)
  (junction 123) -> (junction 141)
  (junction 231) -> (junction 123)
  (junction 141) -> (junction 159)
  data: NtcSts input uint8; Qualifier output uint8 =0; DebStep input uint16; DebCntr local int16

== stateflow chart ES259A_BattVltgCorrln/BattVltgCorrln/BattVltgCorrlnPer1/Battery Voltage Diagnostics/Inhibition Off/BattVltg > OverVltg/SetNtcStsB5/ISO Fault Debounce Design NOT TO BE IMPLEMENTED IN THIS FDD USED ONLY FOR SIMULATION PURPOSES ==
  note: NTCSTS_PASSD           (0)
      | NTCSTS_FAILD             (1)
      | NTCSTS_PREPASSD   (2)
      | NTCSTS_PREFAILD     (3)
      |
      | SIGQLFR_NORES        (0)
      | SIGQLFR_PASSD         (1)
      | SIGQLFR_FAILD           (2)
  note: Fail step Loop
  note: Pass step Loop
  note: 
  (default) -> (junction 89)
  (junction 89) -> (junction 95) [order 1] : [NtcSts == 3]
  (junction 89) -> (junction 93) [order 2] : [ NtcSts == 2]
  (junction 93) -> (junction 230) [order 2] : {
      | DebCntr = DebCntr - DebStep;
      | }
  (junction 95) -> (junction 216) [order 2] : [DebCntr <= 0]
      | {
      | DebCntr = DebStep;
      | }
  (junction 95) -> (junction 103) [order 1] : [DebCntr > 0]
  (junction 93) -> (junction 123) [order 1] : [(DebCntr - DebStep) <= -32768]
      | {
      | DebCntr = -32768;
      | Qualifier = 1;
      | }
  (junction 230) -> (junction 231)
  (junction 103) -> (junction 216) [order 2] : {
      | DebCntr = DebCntr + DebStep;
      | }
  (junction 216) -> (junction 220) [order 2]
  (junction 216) -> (junction 220) [order 1] : [(DebCntr + DebStep) >=32767]
      | {
      | DebCntr = 32767;
      | Qualifier =2;
      | }
  (junction 103) -> (junction 220) [order 1] : [(DebCntr + DebStep) >=32767]
      | {
      | DebCntr = 32767;
      | Qualifier =2;
      | }
  (junction 220) -> (junction 141)
  (junction 123) -> (junction 141)
  (junction 231) -> (junction 123)
  (junction 141) -> (junction 159)
  data: NtcSts input uint8; Qualifier output uint8 =0; DebStep input uint16; DebCntr local int16

== stateflow chart ES259A_BattVltgCorrln/BattVltgCorrln/BattVltgCorrlnPer1/Battery Voltage Diagnostics/Inhibition Off/UnderVltg <= BattVltg < LowVltg/If Action/SetNtcStsB1/ISO Fault Debounce Design NOT TO BE IMPLEMENTED IN THIS FDD USED ONLY FOR SIMULATION PURPOSES ==
  note: NTCSTS_PASSD           (0)
      | NTCSTS_FAILD             (1)
      | NTCSTS_PREPASSD   (2)
      | NTCSTS_PREFAILD     (3)
      |
      | SIGQLFR_NORES        (0)
      | SIGQLFR_PASSD         (1)
      | SIGQLFR_FAILD           (2)
  note: Fail step Loop
  note: Pass step Loop
  note: 
  (default) -> (junction 89)
  (junction 89) -> (junction 95) [order 1] : [NtcSts == 3]
  (junction 89) -> (junction 93) [order 2] : [ NtcSts == 2]
  (junction 93) -> (junction 230) [order 2] : {
      | DebCntr = DebCntr - DebStep;
      | }
  (junction 95) -> (junction 216) [order 2] : [DebCntr <= 0]
      | {
      | DebCntr = DebStep;
      | }
  (junction 95) -> (junction 103) [order 1] : [DebCntr > 0]
  (junction 93) -> (junction 123) [order 1] : [(DebCntr - DebStep) <= -32768]
      | {
      | DebCntr = -32768;
      | Qualifier = 1;
      | }
  (junction 230) -> (junction 231)
  (junction 103) -> (junction 216) [order 2] : {
      | DebCntr = DebCntr + DebStep;
      | }
  (junction 216) -> (junction 220) [order 2]
  (junction 216) -> (junction 220) [order 1] : [(DebCntr + DebStep) >=32767]
      | {
      | DebCntr = 32767;
      | Qualifier =2;
      | }
  (junction 103) -> (junction 220) [order 1] : [(DebCntr + DebStep) >=32767]
      | {
      | DebCntr = 32767;
      | Qualifier =2;
      | }
  (junction 220) -> (junction 141)
  (junction 123) -> (junction 141)
  (junction 231) -> (junction 123)
  (junction 141) -> (junction 159)
  data: NtcSts input uint8; Qualifier output uint8 =0; DebStep input uint16; DebCntr local int16

== stateflow chart ES259A_BattVltgCorrln/BattVltgCorrln/BattVltgCorrlnPer1/Battery Voltage Diagnostics/Inhibition Off/UnderVltg <= BattVltg < LowVltg/If Action/SetNtcStsB5/ISO Fault Debounce Design NOT TO BE IMPLEMENTED IN THIS FDD USED ONLY FOR SIMULATION PURPOSES ==
  note: NTCSTS_PASSD           (0)
      | NTCSTS_FAILD             (1)
      | NTCSTS_PREPASSD   (2)
      | NTCSTS_PREFAILD     (3)
      |
      | SIGQLFR_NORES        (0)
      | SIGQLFR_PASSD         (1)
      | SIGQLFR_FAILD           (2)
  note: Fail step Loop
  note: Pass step Loop
  note: 
  (default) -> (junction 89)
  (junction 89) -> (junction 95) [order 1] : [NtcSts == 3]
  (junction 89) -> (junction 93) [order 2] : [ NtcSts == 2]
  (junction 93) -> (junction 230) [order 2] : {
      | DebCntr = DebCntr - DebStep;
      | }
  (junction 95) -> (junction 216) [order 2] : [DebCntr <= 0]
      | {
      | DebCntr = DebStep;
      | }
  (junction 95) -> (junction 103) [order 1] : [DebCntr > 0]
  (junction 93) -> (junction 123) [order 1] : [(DebCntr - DebStep) <= -32768]
      | {
      | DebCntr = -32768;
      | Qualifier = 1;
      | }
  (junction 230) -> (junction 231)
  (junction 103) -> (junction 216) [order 2] : {
      | DebCntr = DebCntr + DebStep;
      | }
  (junction 216) -> (junction 220) [order 2]
  (junction 216) -> (junction 220) [order 1] : [(DebCntr + DebStep) >=32767]
      | {
      | DebCntr = 32767;
      | Qualifier =2;
      | }
  (junction 103) -> (junction 220) [order 1] : [(DebCntr + DebStep) >=32767]
      | {
      | DebCntr = 32767;
      | Qualifier =2;
      | }
  (junction 220) -> (junction 141)
  (junction 123) -> (junction 141)
  (junction 231) -> (junction 123)
  (junction 141) -> (junction 159)
  data: NtcSts input uint8; Qualifier output uint8 =0; DebStep input uint16; DebCntr local int16

== stateflow chart ES259A_BattVltgCorrln/BattVltgCorrln/BattVltgCorrlnPer1/Battery Voltage Diagnostics/Inhibition Off/UnderVltg <= BattVltg < LowVltg/If Action 1/SetNtcStsB0/ISO Fault Debounce Design NOT TO BE IMPLEMENTED IN THIS FDD USED ONLY FOR SIMULATION PURPOSES ==
  note: NTCSTS_PASSD           (0)
      | NTCSTS_FAILD             (1)
      | NTCSTS_PREPASSD   (2)
      | NTCSTS_PREFAILD     (3)
      |
      | SIGQLFR_NORES        (0)
      | SIGQLFR_PASSD         (1)
      | SIGQLFR_FAILD           (2)
  note: Fail step Loop
  note: Pass step Loop
  note: 
  (default) -> (junction 89)
  (junction 89) -> (junction 95) [order 1] : [NtcSts == 3]
  (junction 89) -> (junction 93) [order 2] : [ NtcSts == 2]
  (junction 93) -> (junction 230) [order 2] : {
      | DebCntr = DebCntr - DebStep;
      | }
  (junction 95) -> (junction 216) [order 2] : [DebCntr <= 0]
      | {
      | DebCntr = DebStep;
      | }
  (junction 95) -> (junction 103) [order 1] : [DebCntr > 0]
  (junction 93) -> (junction 123) [order 1] : [(DebCntr - DebStep) <= -32768]
      | {
      | DebCntr = -32768;
      | Qualifier = 1;
      | }
  (junction 230) -> (junction 231)
  (junction 103) -> (junction 216) [order 2] : {
      | DebCntr = DebCntr + DebStep;
      | }
  (junction 216) -> (junction 220) [order 2]
  (junction 216) -> (junction 220) [order 1] : [(DebCntr + DebStep) >=32767]
      | {
      | DebCntr = 32767;
      | Qualifier =2;
      | }
  (junction 103) -> (junction 220) [order 1] : [(DebCntr + DebStep) >=32767]
      | {
      | DebCntr = 32767;
      | Qualifier =2;
      | }
  (junction 220) -> (junction 141)
  (junction 123) -> (junction 141)
  (junction 231) -> (junction 123)
  (junction 141) -> (junction 159)
  data: NtcSts input uint8; Qualifier output uint8 =0; DebStep input uint16; DebCntr local int16

== stateflow chart ES259A_BattVltgCorrln/BattVltgCorrln/BattVltgCorrlnPer1/Battery Voltage Diagnostics/Inhibition Off/UnderVltg <= BattVltg < LowVltg/If Action 1/SetNtcStsB1/ISO Fault Debounce Design NOT TO BE IMPLEMENTED IN THIS FDD USED ONLY FOR SIMULATION PURPOSES ==
  note: NTCSTS_PASSD           (0)
      | NTCSTS_FAILD             (1)
      | NTCSTS_PREPASSD   (2)
      | NTCSTS_PREFAILD     (3)
      |
      | SIGQLFR_NORES        (0)
      | SIGQLFR_PASSD         (1)
      | SIGQLFR_FAILD           (2)
  note: Fail step Loop
  note: Pass step Loop
  note: 
  (default) -> (junction 89)
  (junction 89) -> (junction 95) [order 1] : [NtcSts == 3]
  (junction 89) -> (junction 93) [order 2] : [ NtcSts == 2]
  (junction 93) -> (junction 230) [order 2] : {
      | DebCntr = DebCntr - DebStep;
      | }
  (junction 95) -> (junction 216) [order 2] : [DebCntr <= 0]
      | {
      | DebCntr = DebStep;
      | }
  (junction 95) -> (junction 103) [order 1] : [DebCntr > 0]
  (junction 93) -> (junction 123) [order 1] : [(DebCntr - DebStep) <= -32768]
      | {
      | DebCntr = -32768;
      | Qualifier = 1;
      | }
  (junction 230) -> (junction 231)
  (junction 103) -> (junction 216) [order 2] : {
      | DebCntr = DebCntr + DebStep;
      | }
  (junction 216) -> (junction 220) [order 2]
  (junction 216) -> (junction 220) [order 1] : [(DebCntr + DebStep) >=32767]
      | {
      | DebCntr = 32767;
      | Qualifier =2;
      | }
  (junction 103) -> (junction 220) [order 1] : [(DebCntr + DebStep) >=32767]
      | {
      | DebCntr = 32767;
      | Qualifier =2;
      | }
  (junction 220) -> (junction 141)
  (junction 123) -> (junction 141)
  (junction 231) -> (junction 123)
  (junction 141) -> (junction 159)
  data: NtcSts input uint8; Qualifier output uint8 =0; DebStep input uint16; DebCntr local int16
